simulink model "random_validate_test"  (R2020b)
settings: Solver=VariableStepAuto  StartTime=0.0  StopTime=10.0  RelTol=1e-3
settings Model: Creator=billy  LastModifiedBy=billy

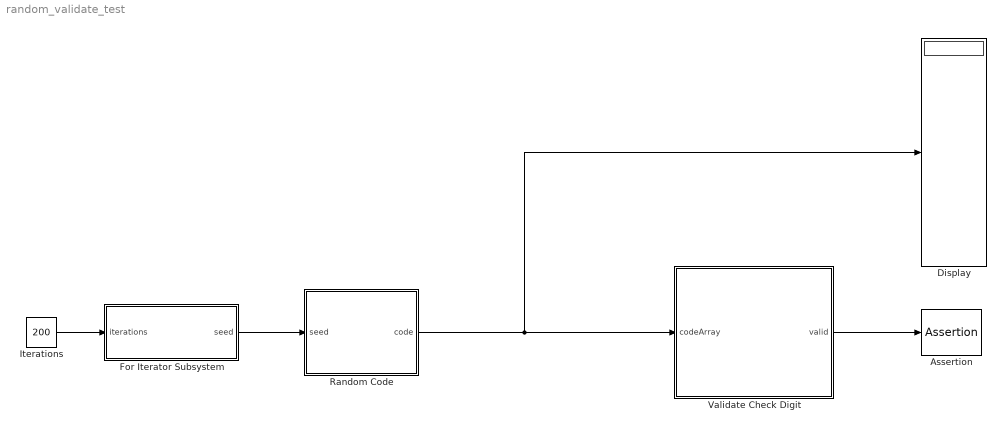
== system random_validate_test ==
  Assertion : Assertion
  Display : Display
  For Iterator Subsystem : Subsystem  TreatAsAtomicUnit=on
  Iterations : Constant  Value=200  OutDataTypeStr=int32
  Random Code : MATLAB Function  TreatAsAtomicUnit=on
  Validate Check Digit : MATLAB Function  TreatAsAtomicUnit=on
  wires:
  Random Code/1(code) -> Validate Check Digit/1(codeArray), Display/1
  For Iterator Subsystem/1(seed) -> Random Code/1(seed)
  Iterations/1 -> For Iterator Subsystem/1(iterations)
  Validate Check Digit/1(valid) -> Assertion/1

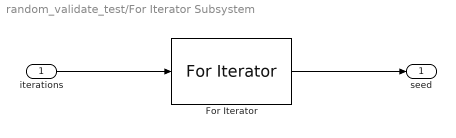
== system random_validate_test/For Iterator Subsystem ==
  iterations : Inport
  For Iterator : ForIterator  IterationSource=external
  seed : Outport
  wires:
  iterations/1 -> For Iterator/1
  For Iterator/1 -> seed/1

== matlab function random_validate_test/Random Code ==
  data: code output size=1,12; seed input
function code = randomupc(seed)
    if(nargin == 1)
        rng(seed);
    end
    
    incompleteCode = incompleteRandomCode();
    digit = calcCheckDigit(incompleteCode);
    code = [incompleteCode digit];
end

function incompleteCode = incompleteRandomCode
    incompleteCode = randi([0,9], 1, 11);
end

function digit = calcCheckDigit(incompleteCode)
    FACTORS = [3; 1; 3; 1; 3; 1; 3; 1; 3; 1; 3];
    m = mod(incompleteCode * FACTORS(1:11), 10);
    
    if(m == 0)
        digit = 0;
    else
        digit = 10 - m;
    end
end

== matlab function random_validate_test/Validate Check Digit ==
  data: codeArray input; valid output
function valid = validateupc(codeArray)
    FACTORS = [3; 1; 3; 1; 3; 1; 3; 1; 3; 1; 3; 1];
    valid = mod(codeArray * FACTORS, 10) == 0;
end
